simulink model "gain"  (Simulink 7.3)
settings: Solver=FixedStepDiscrete  StartTime=0.0  StopTime=10.0  FixedStep=1  RelTol=1e-3
settings Model: Creator=ksmyth  LastModifiedBy=hnine
settings DataIOCC: SaveFormat=Structure
settings OptimizationCC: InitFltsAndDblsToZero=on
settings DebuggingCC: SaveWithParameterizedLinksMsg=none
settings GRTTargetCC: TargetFcnLib=ansi_tfl_tmw.mat

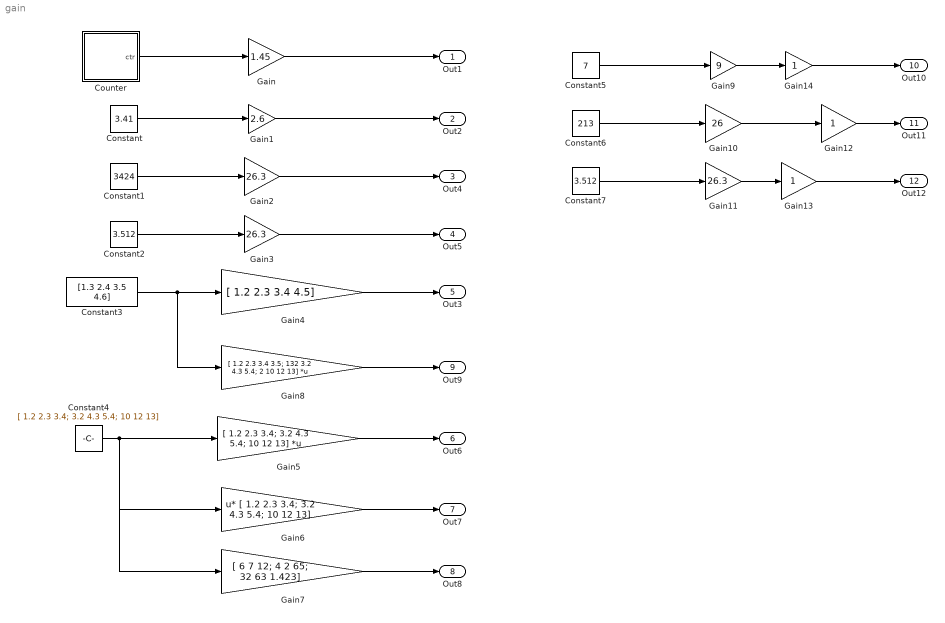
== system gain ==
  Constant : Constant  Value=3.41  OutDataTypeMode=double  OutDataType=sfix(16)  OutScaling=2^0  OutDataTypeStr=double
  Constant1 : Constant  Value=3424  OutDataTypeMode=uint16  OutDataType=sfix(16)  OutScaling=2^0  OutDataTypeStr=uint16
  Constant2 : Constant  Value=3.512  OutDataTypeMode=double  OutDataType=sfix(16)  OutScaling=2^0  OutDataTypeStr=double
  Constant3 : Constant  Value=[1.3 2.4 3.5 4.6]  OutDataTypeMode=double  OutDataType=sfix(16)  OutScaling=2^0  OutDataTypeStr=double
  Constant4 : Constant  Value=[ 1.2 2.3 3.4; 3.2 4.3 5.4; 10 12 13]  OutDataType=sfix(16)  OutScaling=2^0
  Constant5 : Constant  Value=7  OutDataTypeMode=int32  OutDataType=sfix(16)  OutScaling=2^0  OutDataTypeStr=int32
  Constant6 : Constant  Value=213  OutDataTypeMode=uint8  OutDataType=sfix(16)  OutScaling=2^0  OutDataTypeStr=uint8
  Constant7 : Constant  Value=3.512  OutDataTypeMode=double  OutDataType=sfix(16)  OutScaling=2^0  OutDataTypeStr=double
  Counter : Stateflow chart
  Gain : Gain  Gain=1.45  ParameterDataType=sfix(16)  ParameterScaling=2^0  OutDataType=sfix(16)  OutScaling=2^0
  Gain1 : Gain  Gain=2.6  ParameterDataType=sfix(16)  ParameterScaling=2^0  OutDataType=sfix(16)  OutScaling=2^0
  Gain10 : Gain  Gain=26  ParameterDataType=float('single')  ParameterScaling=2^0  OutDataType=float('double')  OutScaling=2^0
  Gain11 : Gain  Gain=26.3  ParameterDataTypeMode=Specify via dialog  ParameterDataType=float('double')  ParameterScaling=2^0  ParamDataTypeStr=float('double')  OutDataTypeMode=Specify via dialog  OutDataType=float('double')  OutScaling=2^0  OutDataTypeStr=float('double')
  Gain12 : Gain  ParameterDataTypeMode=Specify via dialog  ParameterDataType=float('single')  ParameterScaling=2^0  ParamDataTypeStr=float('single')  OutDataTypeMode=Specify via dialog  OutDataType=float('double')  OutScaling=2^0  OutDataTypeStr=float('double')
  Gain13 : Gain  ParameterDataTypeMode=Specify via dialog  ParameterDataType=float('double')  ParameterScaling=2^0  ParamDataTypeStr=float('double')  OutDataTypeMode=Specify via dialog  OutDataType=float('double')  OutScaling=2^0  OutDataTypeStr=float('double')
  Gain14 : Gain  ParameterDataType=sfix(16)  ParameterScaling=2^0  OutDataTypeMode=Specify via dialog  OutDataType=float('double')  OutScaling=2^0  OutDataTypeStr=float('double')
  Gain2 : Gain  Gain=26.3  ParameterDataTypeMode=Specify via dialog  ParameterDataType=float('double')  ParameterScaling=2^0  ParamDataTypeStr=float('double')  OutDataTypeMode=Specify via dialog  OutDataType=float('double')  OutScaling=2^0  OutDataTypeStr=float('double')
  Gain3 : Gain  Gain=26.3  ParameterDataTypeMode=Specify via dialog  ParameterDataType=float('double')  ParameterScaling=2^0  ParamDataTypeStr=float('double')  OutDataTypeMode=Specify via dialog  OutDataType=float('double')  OutScaling=2^0  OutDataTypeStr=float('double')
  Gain4 : Gain  Gain=[ 1.2 2.3 3.4 4.5]  ParameterDataType=sfix(16)  ParameterScaling=2^0  OutDataType=float('double')  OutScaling=2^0  OutDataTypeStr=Inherit: Same as input
  Gain5 : Gain  Gain=[ 1.2 2.3 3.4; 3.2 4.3 5.4; 10 12 13]  Multiplication=Matrix(K*u)  ParameterDataType=sfix(16)  ParameterScaling=2^0  OutDataType=float('double')  OutScaling=2^0  OutDataTypeStr=Inherit: Same as input
  Gain6 : Gain  Gain=[ 1.2 2.3 3.4; 3.2 4.3 5.4; 10 12 13]  Multiplication=Matrix(u*K)  ParameterDataType=sfix(16)  ParameterScaling=2^0  OutDataType=float('double')  OutScaling=2^0  OutDataTypeStr=Inherit: Same as input
  Gain7 : Gain  Gain=[ 6 7 12; 4 2 65; 32 63 1.423]  ParameterDataType=sfix(16)  ParameterScaling=2^0  OutDataType=float('double')  OutScaling=2^0  OutDataTypeStr=Inherit: Same as input
  Gain8 : Gain  Gain=[ 1.2 2.3 3.4 3.5; 132 3.2 4.3 5.4; 2 10 12 13]  Multiplication=Matrix(K*u) (u vector)  ParameterDataType=sfix(16)  ParameterScaling=2^0  OutDataType=float('double')  OutScaling=2^0  OutDataTypeStr=Inherit: Same as input
  Gain9 : Gain  Gain=9  ParameterDataType=sfix(16)  ParameterScaling=2^0  OutDataType=sfix(16)  OutScaling=2^0  OutDataTypeStr=Inherit: Same as input
  Out1 : Outport  OutDataType=sfix(16)  OutScaling=2^0
  Out2 : Outport  Port=2  OutDataType=sfix(16)  OutScaling=2^0
  Out4 : Outport  Port=3  OutDataType=sfix(16)  OutScaling=2^0
  Out5 : Outport  Port=4  OutDataType=sfix(16)  OutScaling=2^0
  Out3 : Outport  Port=5  OutDataType=sfix(16)  OutScaling=2^0
  Out6 : Outport  Port=6  OutDataType=sfix(16)  OutScaling=2^0
  Out7 : Outport  Port=7  OutDataType=sfix(16)  OutScaling=2^0
  Out8 : Outport  Port=8  OutDataType=sfix(16)  OutScaling=2^0
  Out9 : Outport  Port=9  OutDataType=sfix(16)  OutScaling=2^0
  Out10 : Outport  Port=10  OutDataType=sfix(16)  OutScaling=2^0
  Out11 : Outport  Port=11  OutDataType=sfix(16)  OutScaling=2^0
  Out12 : Outport  Port=12  OutDataType=sfix(16)  OutScaling=2^0
  wires:
  Counter/1(ctr) -> Gain/1
  Gain/1 -> Out1/1
  Constant/1 -> Gain1/1
  Gain1/1 -> Out2/1
  Constant1/1 -> Gain2/1
  Constant2/1 -> Gain3/1
  Gain2/1 -> Out4/1
  Gain3/1 -> Out5/1
  Constant3/1 -> Gain4/1, Gain8/1
  Gain4/1 -> Out3/1
  Gain5/1 -> Out6/1
  Constant4/1 -> Gain5/1, Gain6/1, Gain7/1
  Gain6/1 -> Out7/1
  Gain7/1 -> Out8/1
  Gain8/1 -> Out9/1
  Constant5/1 -> Gain9/1
  Constant6/1 -> Gain10/1
  Constant7/1 -> Gain11/1
  Gain9/1 -> Gain14/1
  Gain14/1 -> Out10/1
  Gain10/1 -> Gain12/1
  Gain12/1 -> Out11/1
  Gain11/1 -> Gain13/1
  Gain13/1 -> Out12/1

== stateflow chart Counter ==
  state s1
  (default) -> s1
  s1 -> s1 [order 1] : [ctr < 4] / ctr = ctr+1;
  s1 -> s1 [order 2] : [ctr >= 4] / ctr = 0;
  data: ctr output double =1
